simulink model "test_r2_butterfly_j"  (Simulink 6.2)
settings: Solver=ode45  StartTime=0.0  StopTime=10.0  RelTol=1e-3
libraries: xbsIndex_r3 x7
settings Model: LastModifiedBy=mdexter
settings DebuggingCC: SolverPrmCheckMsg=warning

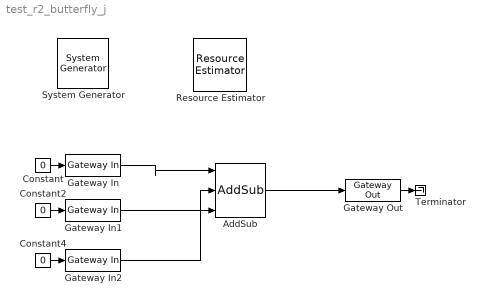
== system test_r2_butterfly_j ==
  " System Generator" : xbsIndex_r3/ System Generator  Tag=genX  xilinxfamily=Virtex2  part=xc2v1000  speed=-4  package=bg575  synthesis_tool=XST  directory=./netlist  testbench=off  simulink_period=1  sysclk_period=100  incr_netlist=off  trim_vbits=Everywhere in SubSystem  dbl_ovrd=According to Block Masks  core_generation=According to Block Masks  run_coregen=off  deprecated_control=off  eval_field=0
      settings: AttributesFormatString=System\nGenerator
  AddSub : xbsIndex_r3/AddSub  mode=Addition or Subtraction  precision=Full  arith_type=Unsigned  n_bits=8  bin_pt=2  quantization=Truncate  overflow=Wrap  latency=1  explicit_period=off  period=1  use_carryin=off  use_carryout=off  en=off  dbl_ovrd=off  show_param=on  use_core=on  pipeline=on  use_rpm=on  gen_core=off
      settings: xl_area=[5 9 0 9 0 0 0]
  Constant : Constant  Value=0
  Constant2 : Constant  Value=0
  Constant4 : Constant  Value=0
  Gateway In : xbsIndex_r3/Gateway In  arith_type="Signed  (2's comp)"  n_bits=8  bin_pt=7  quantization=Truncate  overflow=Wrap  period=1  timing_constraint=None  locs_specified=off  LOCs={}  needs_fixed_name=off  dbl_ovrd=off  show_param=off
      settings: xl_area=[0 0 0 0 8 0 0]
  Gateway In1 : xbsIndex_r3/Gateway In  arith_type="Signed  (2's comp)"  n_bits=8  bin_pt=7  quantization=Truncate  overflow=Wrap  period=1  timing_constraint=None  locs_specified=off  LOCs={}  needs_fixed_name=off  dbl_ovrd=off  show_param=off
      settings: xl_area=[0 0 0 0 8 0 0]
  Gateway In2 : xbsIndex_r3/Gateway In  arith_type=Boolean  n_bits=8  bin_pt=7  quantization=Truncate  overflow=Wrap  period=1  timing_constraint=None  locs_specified=off  LOCs={}  needs_fixed_name=off  dbl_ovrd=off  show_param=off
      settings: xl_area=[0 0 0 0 1 0 0]
  Gateway Out : xbsIndex_r3/Gateway Out  output_type=Double  nbits=8  bin_pt=6  arith_type=Boolean  quantization=Truncate  overflow=Wrap  hdl_port=on  timing_constraint=None  locs_specified=off  LOCs={}  needs_fixed_name=off  show_param=off
      settings: xl_area=[0 0 0 0 9 0 0]
  Resource Estimator : xbsIndex_r3/Resource Estimator  Tag=resEstTag  xl_estimator_area=[5 9 0 9 26 0 0]  xl_use_estimator_area=off  simulink_period=1  mrp_directory=./netlist
      settings: AttributesFormatString=Resource Estimator\n%<xl_estimator_area>\n[SL FF BR LUT IO MUL TBUF]
  Terminator : Terminator
  wires:
  Gateway In/1 -> AddSub/1
  AddSub/1 -> Gateway Out/1
  Constant/1 -> Gateway In/1
  Constant2/1 -> Gateway In1/1
  Gateway Out/1 -> Terminator/1
  Constant4/1 -> Gateway In2/1
  Gateway In2/1 -> AddSub/3
  Gateway In1/1 -> AddSub/2
